simulink model "Motore_11_MM2"  (R2023b)
settings: Solver=ode23tb  StartTime=0.0  StopTime=193  FixedStep=0.001  MaxStep=1e-4  RelTol=1e-3  AbsTol=1e-2
InitFcn:
  | %Matrice=readmatrix('Profilo.csv');
  | clear
  | clc
  | 
  | m_bike=10;
  | m_driver=75;
  | mass=m_bike+m_driver;
  | a=1;
  | b=0.8;
  | h=1;
  | R=0.33;
  | 
  | load("Map.mat")
  | load("VSOC2.mat")
  | load("DriveCycle.mat")
  | t1=DriveCycle(:,1);
  | v1=DriveCycle(:,2);
  | x=length(t1);
  | t1(x)=[];
  | v1(x)=[];
  | 
  | voltage=flip(VSOC2(:,2));
  | SOC=flip(VSOC2(:,1))/100;
  | 
  | v=Map(:,1);
  | v=v*1000/3600;
  | 
  | w=v/R;
  | w=w';
  | T=Map(:,2);
  | T=T';
  | 
  | Np=1;
  | Ns=10;
  | Capacity=2; % Ah
  | 
  | k_trasm=2;
undefined symbols (not defined in the file): Map
libraries: simulink x7, slpidlib x4, autolibshared x1
settings Model: Creator=fabio  LastModifiedBy=marce
settings SolverCC: ZeroCrossAlgorithm=Adaptive
settings OptimizationCC: ReuseModelBlockBuffer=off
settings DebuggingCC: IgnoredZcDiagnostic=none

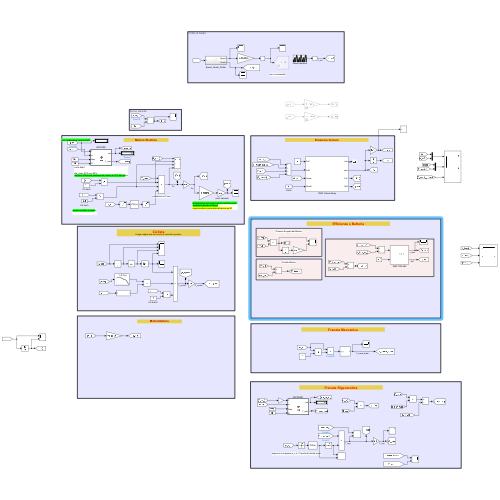
[thumbnail: Simulink's stored preview of the top-level diagram]
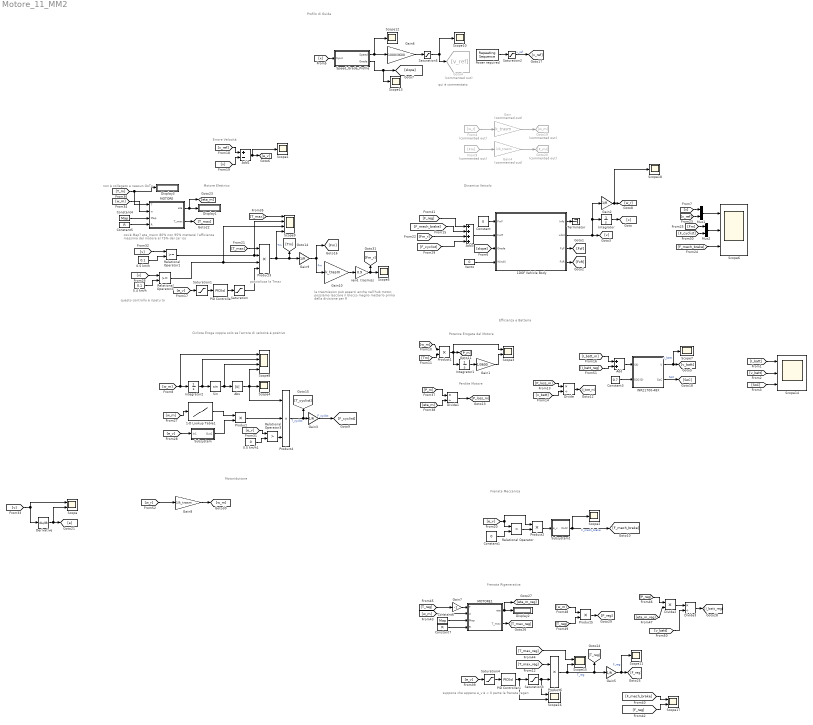
== system Motore_11_MM2 ==
  note: suppone che appena e_v è < 0 parte la frenata regen
  note: parzializza la Tmax
  note: non è collegato a neesun GoTo
  note: qui è commentato
  note: la trasmission può esserci anche nell'hub motor,
      | possiamo lasciare il blocco
      | meglio metterlo prima della divisione per R
  note: cos'è Map?
      |
      | eta_max= 80% non 95%
      | metterei l'efficienza massima del motore al 75% del car ico
  note: questo controllo è ripetu to
  note: Potenza Erogata dal Motore
  note: Motore Elettrico
  note: Profilo di Guida
  note: Errore Velocità
  note: Ciclista
      | Eroga coppia solo se l'errore di velocità è positivo
  note: Efficienza e Batteria
  note: Dinamica Veicolo
  note: Perdite Motore
  note: Frenata Rigenerativa
  note: Frenata Meccanica
  note: Motoriduttore
  " INR21700-48X" : Subsystem
      mask Display: image('C:\Users\fabio\OneDrive\Desktop\Screenshot 2023-04-19 143832.png'); % Use "Edit Image" on toolstrip to change.
  0.5 km/h : Constant  Value=0.1
  0.5 km/h1 : Constant  Value=0
  1-D Lookup Table1 : Lookup_n-D  NumberOfTableDimensions=1  BreakpointsForDimension1=w  Table=T  InternalRulePriority=Speed  RndMeth=Simplest
  1DOF Vehicle Body : Subsystem
  5.4 km/h : Constant  Value=0.1
  Abs : Abs  SaturateOnIntegerOverflow=off
  Add : Sum
  Add1 : Sum  Inputs=+-
  Add3 : Sum  Inputs=++++
  Constant : Constant  Value=0
  Constant1 : Constant  Value=0
  Constant3 : Constant  Value=0.7
  Constant4 : Constant  Value=Map
  Constant5 : Constant  Value=R
  Constant6 : Constant  Value=Map
  Constant7 : Constant  Value=R
  Derivative : Derivative
  Display1 : Display
  Display2 : Display
  Display3 : Display
  Divide : Product  Inputs=*/
  Divide1 : Product  Inputs=*/
  Divide2 : Product  Inputs=**
  Divide3 : Product  Inputs=*/
  From4 : From  Commented=on  GotoTag=w_r
  From9 : From  Commented=on  GotoTag=Fm
  Gain : Gain  Commented=on  Gain=k_trasm
  Gain1 : Gain  Gain=1/3600
  Gain10 : Gain  Gain=k_trasm
  Gain{2..3,5,9} (4 alike) : Gain  Gain=1/R
  Gain4 : Gain  Commented=on  Gain=1/k_trasm
  Gain6 : Gain  Gain=1000/3600
  Gain7 : Gain  Gain=-1
  Gain8 : Gain  Gain=1/k_trasm
  Goto19 : Goto  Commented=on  GotoTag=w_m
  Goto20 : Goto  Commented=on  GotoTag=F_mr
  Goto4 : Goto  Commented=on  GotoTag=v_ref
  Integrator : Integrator
  Integrator1 : Integrator
  Integrator2 : Integrator
  MOTORE : MATLAB Function  TreatAsAtomicUnit=on
  MOTORE1 : MATLAB Function  TreatAsAtomicUnit=on
  Mux1 : Mux  Inputs=2
  Mux2 : Mux  Inputs=2
  PID Controller : slpidlib/PID Controller  Controller=PID  Form=Parallel  TimeDomain=Continuous-time  UseExternalTs=off  SampleTime=-1  IntegratorMethod=Forward Euler  FilterMethod=Forward Euler  ControllerParametersSource=internal  P=5  I=0  UseKiTs=off  D=0  N=100  UseFilter=on  TunerSelectOption=Transfer Function Based (PID Tuner App)  InitialConditionSource=internal  InitialConditionForIntegrator=0  InitialConditionForFilter=0  DifferentiatorICPrevScaledInput=0  ExternalReset=none  TrackingMode=off  Kt=1  LimitOutput=off  SatLimitsSource=internal  UpperSaturationLimit=inf  LowerSaturationLimit=-inf  LinearizeAsGain=on  AntiWindupMode=none  Kb=1  LimitIntegrator=off  UpperIntegratorSaturationLimit=inf  LowerIntegratorSaturationLimit=-inf  POutMin=[]  POutMax=[]  IOutMin=[]  IOutMax=[]  DOutMin=[]  DOutMax=[]  NOutMin=[]  NOutMax=[]  SumOutMin=[]  SumOutMax=[]  SaturationOutMin=[]  SaturationOutMax=[]  PParamMin=[]  PParamMax=[]  IParamMin=[]  IParamMax=[]  DParamMin=[]  DParamMax=[]  NParamMin=[]  NParamMax=[]  KbParamMin=[]  KbParamMax=[]  KtParamMin=[]  KtParamMax=[]  KbOutMin=[]  KbOutMax=[]  KtOutMin=[]  KtOutMax=[]  IntegratorOutMin=[]  IntegratorOutMax=[]  FilterOutMin=[]  FilterOutMax=[]  SumI1OutMin=[]  SumI1OutMax=[]  SumI2OutMin=[]  SumI2OutMax=[]  SumI3OutMin=[]  SumI3OutMax=[]  SumI4OutMin=[]  SumI4OutMax=[]  SumDOutMin=[]  SumDOutMax=[]  DifferentiatorOutMin=[]  DifferentiatorOutMax=[]  FilterDiffOutCoefMin=[]  FilterDiffOutCoefMax=[]  ReciprocalOutMin=[]  ReciprocalOutMax=[]  SumDenOutMin=[]  SumDenOutMax=[]  SumNumOutMin=[]  SumNumOutMax=[]  DivideOutMin=[]  DivideOutMax=[]  UdiffTsProdOutMin=[]  UdiffTsProdOutMax=[]  NTsProdOutMin=[]  NTsProdOutMax=[]  UintegralTsProdOutMin=[]  UintegralTsProdOutMax=[]  UngainTsProdOutMin=[]  UngainTsProdOutMax=[]  ClampingZeroOutDataTypeStr=Inherit: Inherit via back propagation  ClampingZeroOutMin=[]  ClampingZeroOutMax=[]  FilterDenConstantOutDataTypeStr=Inherit: Inherit via back propagation  FilterDenConstantOutMin=[]  FilterDenConstantOutMax=[]  PCopyOutDataTypeStr=Inherit: Inherit via back propagation  PCopyOutMin=[]  PCopyOutMax=[]  NCopyOutDataTypeStr=Inherit: Inherit via back propagation  NCopyOutMin=[]  NCopyOutMax=[]  IntegratorContinuousStateAttributes=''  IntegratorStateMustResolveToSignalObject=off  IntegratorRTWStateStorageClass=Auto  FilterContinuousStateAttributes=''  FilterStateMustResolveToSignalObject=off  FilterRTWStateStorageClass=Auto  ParallelPVariant=InternalParameters  IdealPVariant=Disabled  IVariant=InternalParameters  DVariant=InternalParameters  IntegratorVariant=Continuous  SatVariant=Disabled  AWVariant=Passthrough  PCopyVariant=Disabled  TRVariant=Disabled  FdbkBlocksVariant=Forward  IdealPFdbkVariant=Disabled  SatFdbkVariant=Disabled  DerivativeFilterVariant=ContFilter  NVariant=InternalParameters  NCopyVariant=Disabled  FilterICVariant=InternalICsFilter  IntegratorICVariant=InternalICs  ExternalResetVariant=Disabled  TRSumVariant=Passthrough  SumFdbkVariant=Disabled  SumVariant=Sum_PID  TsampFilterVariant=InternalTs  TsampNgainVariant=Passthrough  TsampIntegralVariant=Disabled_SignalSpec  ExternalSaturationOutDataTypeStr=Inherit: Same as second input
  PID Controller1 : slpidlib/PID Controller  Controller=PID  Form=Parallel  TimeDomain=Continuous-time  UseExternalTs=off  SampleTime=-1  IntegratorMethod=Forward Euler  FilterMethod=Forward Euler  ControllerParametersSource=internal  P=5000  I=0  UseKiTs=off  D=0  N=100  UseFilter=on  TunerSelectOption=Transfer Function Based (PID Tuner App)  InitialConditionSource=internal  InitialConditionForIntegrator=0  InitialConditionForFilter=0  DifferentiatorICPrevScaledInput=0  ExternalReset=none  TrackingMode=off  Kt=1  LimitOutput=off  SatLimitsSource=internal  UpperSaturationLimit=inf  LowerSaturationLimit=-inf  LinearizeAsGain=on  AntiWindupMode=none  Kb=1  LimitIntegrator=off  UpperIntegratorSaturationLimit=inf  LowerIntegratorSaturationLimit=-inf  POutMin=[]  POutMax=[]  IOutMin=[]  IOutMax=[]  DOutMin=[]  DOutMax=[]  NOutMin=[]  NOutMax=[]  SumOutMin=[]  SumOutMax=[]  SaturationOutMin=[]  SaturationOutMax=[]  PParamMin=[]  PParamMax=[]  IParamMin=[]  IParamMax=[]  DParamMin=[]  DParamMax=[]  NParamMin=[]  NParamMax=[]  KbParamMin=[]  KbParamMax=[]  KtParamMin=[]  KtParamMax=[]  KbOutMin=[]  KbOutMax=[]  KtOutMin=[]  KtOutMax=[]  IntegratorOutMin=[]  IntegratorOutMax=[]  FilterOutMin=[]  FilterOutMax=[]  SumI1OutMin=[]  SumI1OutMax=[]  SumI2OutMin=[]  SumI2OutMax=[]  SumI3OutMin=[]  SumI3OutMax=[]  SumI4OutMin=[]  SumI4OutMax=[]  SumDOutMin=[]  SumDOutMax=[]  DifferentiatorOutMin=[]  DifferentiatorOutMax=[]  FilterDiffOutCoefMin=[]  FilterDiffOutCoefMax=[]  ReciprocalOutMin=[]  ReciprocalOutMax=[]  SumDenOutMin=[]  SumDenOutMax=[]  SumNumOutMin=[]  SumNumOutMax=[]  DivideOutMin=[]  DivideOutMax=[]  UdiffTsProdOutMin=[]  UdiffTsProdOutMax=[]  NTsProdOutMin=[]  NTsProdOutMax=[]  UintegralTsProdOutMin=[]  UintegralTsProdOutMax=[]  UngainTsProdOutMin=[]  UngainTsProdOutMax=[]  ClampingZeroOutDataTypeStr=Inherit: Inherit via back propagation  ClampingZeroOutMin=[]  ClampingZeroOutMax=[]  FilterDenConstantOutDataTypeStr=Inherit: Inherit via back propagation  FilterDenConstantOutMin=[]  FilterDenConstantOutMax=[]  PCopyOutDataTypeStr=Inherit: Inherit via back propagation  PCopyOutMin=[]  PCopyOutMax=[]  NCopyOutDataTypeStr=Inherit: Inherit via back propagation  NCopyOutMin=[]  NCopyOutMax=[]  IntegratorContinuousStateAttributes=''  IntegratorStateMustResolveToSignalObject=off  IntegratorRTWStateStorageClass=Auto  FilterContinuousStateAttributes=''  FilterStateMustResolveToSignalObject=off  FilterRTWStateStorageClass=Auto  ParallelPVariant=InternalParameters  IdealPVariant=Disabled  IVariant=InternalParameters  DVariant=InternalParameters  IntegratorVariant=Continuous  SatVariant=Disabled  AWVariant=Passthrough  PCopyVariant=Disabled  TRVariant=Disabled  FdbkBlocksVariant=Forward  IdealPFdbkVariant=Disabled  SatFdbkVariant=Disabled  DerivativeFilterVariant=ContFilter  NVariant=InternalParameters  NCopyVariant=Disabled  FilterICVariant=InternalICsFilter  IntegratorICVariant=InternalICs  ExternalResetVariant=Disabled  TRSumVariant=Passthrough  SumFdbkVariant=Disabled  SumVariant=Sum_PID  TsampFilterVariant=InternalTs  TsampNgainVariant=Passthrough  TsampIntegralVariant=Disabled_SignalSpec  ExternalSaturationOutDataTypeStr=Inherit: Same as second input
  Power required : simulink/Sources/Repeating Sequence  rep_seq_t=t1  rep_seq_y=v1
  Product{,1..2,5..6} (5 alike) : Product
  Product3 : Product  Inputs=4
  Product4 : Product  Inputs=3
  Relational Operator : RelationalOperator  Operator=<  OutDataTypeStr=boolean  RndMeth=Simplest  InputSameDT=off
  Relational Operator1 : RelationalOperator  OutDataTypeStr=boolean  RndMeth=Simplest  InputSameDT=off
  Relational Operator2 : RelationalOperator  OutDataTypeStr=boolean  RndMeth=Simplest  InputSameDT=off
  Relational Operator3 : RelationalOperator  Operator=>  OutDataTypeStr=boolean  RndMeth=Simplest  InputSameDT=off
  Saturation : Saturate  UpperLimit=1  LowerLimit=0
  Saturation1 : Saturate  UpperLimit=inf  LowerLimit=0
  Saturation2 : Saturate  UpperLimit=inf  LowerLimit=0
  Saturation3 : Saturate  UpperLimit=0  LowerLimit=-1
  Saturation4 : Saturate  UpperLimit=0  LowerLimit=-inf
  Saturation5 : Saturate  UpperLimit=inf  LowerLimit=0
  Scope{,3,15..17} (5 alike) : Scope  NumInputPorts=2
  Scope{1..2,4..5,7,10..13,18} (10 alike) : Scope
  Scope14 : Scope  NumInputPorts=3
  Scope6 : Scope  NumInputPorts=3
  Scope8 : Scope  NumInputPorts=4
  Scope9 : Scope  NumInputPorts=4
  Sin : Trigonometry
  Speed_Grade_Profile : Subsystem
  Subsystem : Subsystem
  Subsystem1 : Subsystem
  Terminator : Terminator
  Vento : Constant  Value=0
  rend. trasmiss : Gain  Gain=0.9
  wires:
  Vento/1 -> 1DOF Vehicle Body/4(WindX)
  1DOF Vehicle Body/1(Info) -> Terminator/1
  Integrator/1 -> [x]
  1DOF Vehicle Body/4(FzR) -> [FzR]
  1DOF Vehicle Body/3(FzF) -> [Fzf]
  1DOF Vehicle Body/2(xdot) -> Gain2/1, Integrator/1, [v]
  [slope] -> 1DOF Vehicle Body/3(Grade)
  Speed_Grade_Profile/2(Grade) -> Scope13/1, [slope]
  [x] -> Speed_Grade_Profile/1(Input)
  Speed_Grade_Profile/1(Speed) -> Scope12/1, Gain6/1
  Gain6/1 -> Saturation5/1
  Saturation5/1 -> Scope10/1, Goto4/1
  Add3/1 -> 1DOF Vehicle Body/2(FwR)
  [P_loss_m] -> Divide/1
  [v_batt] -> Divide/2
  Divide/1 -> [I_batt_m]
  Constant3/1 -> " INR21700-48X"/2(SOC(0))
  " INR21700-48X"/1(V) -> Scope7/1, [v_batt]  "v_batt"
  Constant/1 -> 1DOF Vehicle Body/1(FwF)
  [v] -> Add1/2
  [v_ref] -> Add1/1
  Add1/1 -> Scope1/1, [e_v]
  Constant1/1 -> Relational Operator/2
  [e_v] -> Product2/1, Relational Operator/1
  Relational Operator/1 -> Product2/2
  Product2/1 -> Subsystem1/1(e_v)
  Subsystem1/1(Out2) -> Scope2/1, [F_mech_brake]  "F_mech_brake"
  [e_v] -> Saturation1/1
  0.5 km/h/1 -> Relational Operator1/2
  Gain9/1 -> Gain10/1, [Fm]  "Fm"
  [w_m] -> Scope8/1, Integrator2/1
  Integrator2/1 -> Scope8/2, Sin/1
  Sin/1 -> Scope8/3, Abs/1
  Abs/1 -> Scope8/4, Product4/1, Scope4/1
  [v] -> Mux1/1
  Mux1/1 -> Scope6/1
  [v_ref] -> Mux1/2
  Mux2/1 -> Scope6/2
  Gain2/1 -> Scope18/1, [w_r]
  [v] -> Relational Operator2/1
  5.4 km/h/1 -> Relational Operator2/2
  Relational Operator2/1 -> Scope9/3, Product3/3
  [w_m] -> 1-D Lookup Table1/1
  1-D Lookup Table1/1 -> Product/1
  Subsystem/1(Out1) -> Product/2
  [e_v] -> Subsystem/1(In1)
  Product/1 -> Product4/2
  Product4/1 -> [T_cyclist], Gain3/1  "T_cyclist"
  Gain3/1 -> [F_cyclist]  "F_cyclist"
  [F_cyclist] -> Mux2/2
  [Fm] -> Mux2/1
  [F_mech_brake] -> Scope6/3
  Product3/1 -> Scope9/4, Gain9/1, [Tm]  "Tm"
  [e_v] -> Relational Operator3/1
  0.5 km/h1/1 -> Relational Operator3/2
  Relational Operator3/1 -> Product4/3
  Gain1/1 -> Scope3/2
  [w_m] -> Product1/1
  Product1/1 -> Scope3/1, [P_m], Integrator1/1
  [Tm] -> Product1/2
  Integrator1/1 -> Gain1/1
  [I_batt] -> Scope14/1
  [v_batt] -> Scope14/2
  " INR21700-48X"/2(SoC) -> [SoC]  "SoC"
  [SoC] -> Scope14/3
  Relational Operator1/1 -> Scope9/2, Product3/2
  From4/1 -> Gain/1
  Gain/1 -> Goto19/1
  From9/1 -> Gain4/1
  Gain4/1 -> Goto20/1
  PID Controller/1 -> Saturation/1
  [v] -> Relational Operator1/1
  Saturation1/1 -> PID Controller/1
  Saturation/1 -> Product3/4
  Power required/1 -> Saturation2/1
  Saturation2/1 -> [v_ref]  "v_ref"
  [v] -> Scope/1, Derivative/1
  Derivative/1 -> Scope/2, [a]
  [w_m] -> MOTORE/2(w)
  MOTORE/1(eta) -> [eta_m], Display1/1
  Constant4/1 -> MOTORE/3(Map)
  Constant5/1 -> MOTORE/4(R)
  MOTORE/2(T_max) -> [T_max]
  [T_max] -> Product3/1
  [T_max] -> Scope9/1
  [T_m] -> MOTORE/1(T), Display3/1
  [P_m] -> Divide1/1
  [eta_m] -> Divide1/2
  Divide1/1 -> [P_loss_m]
  Gain5/1 -> Scope11/1, [F_reg]  "F_reg"
  [T_max_reg] -> Scope15/1
  Saturation3/1 -> Scope16/1, Product6/2
  PID Controller1/1 -> Scope16/2, Saturation3/1
  [T_max_reg] -> Product6/1
  MOTORE1/2(T_max) -> [T_max_reg]
  [e_v] -> Saturation4/1
  MOTORE1/1(eta) -> [eta_m_reg], Display2/1
  Saturation4/1 -> PID Controller1/1
  [T_reg] -> Gain7/1
  Constant7/1 -> MOTORE1/4(R)
  Constant6/1 -> MOTORE1/3(Map)
  [w_m] -> MOTORE1/2(w)
  [F_cyclist] -> Add3/4
  [Fm_r] -> Add3/3
  [F_mech_brake] -> Add3/2
  [F_reg] -> Add3/1
  Product6/1 -> Scope15/2, [T_reg], Gain5/1  "T_reg"
  Gain7/1 -> MOTORE1/1(T)
  [F_mech_brake] -> Scope17/1
  [F_reg] -> Scope17/2
  Divide2/1 -> Divide3/1
  [eta_m_reg] -> Divide2/2
  [P_reg] -> Divide2/1
  Product5/1 -> [P_reg]
  [w_m] -> Product5/1
  [T_reg] -> Product5/2
  [v_batt] -> Divide3/2
  Divide3/1 -> [I_batt_reg]
  Add/1 -> " INR21700-48X"/1(I(A))
  [I_batt_m] -> Add/1
  [I_batt_reg] -> Add/2
  [w_r] -> Gain8/1
  Gain8/1 -> [w_m]
  Gain10/1 -> rend. trasmiss/1
  rend. trasmiss/1 -> [Fm_r], Scope5/1

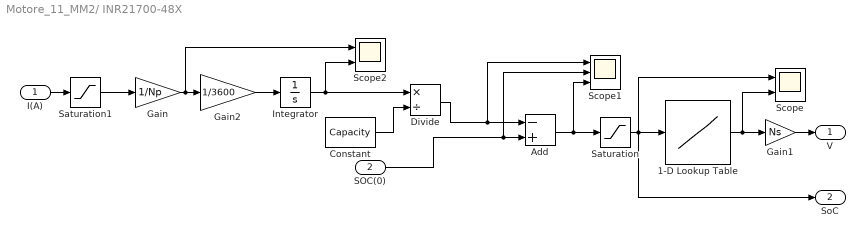
== system Motore_11_MM2/ INR21700-48X ==
  I(A) : Inport
  SOC(0) : Inport  Port=2
  1-D Lookup Table : Lookup_n-D  NumberOfTableDimensions=1  BreakpointsForDimension1=SOC  Table=voltage  InternalRulePriority=Speed  RndMeth=Simplest
  Add : Sum  Inputs=-+
  Constant : Constant  Value=Capacity
  Divide : Product  Inputs=*/
  Gain : Gain  Gain=1/Np
  Gain1 : Gain  Gain=Ns
  Gain2 : Gain  Gain=1/3600
  Integrator : Integrator
  Saturation : Saturate  UpperLimit=1  LowerLimit=0
  Saturation1 : Saturate  UpperLimit=1e6  LowerLimit=-1e6
  Scope : Scope  NumInputPorts=2
  Scope1 : Scope  NumInputPorts=3
  Scope2 : Scope  NumInputPorts=2
  V : Outport
  SoC : Outport  Port=2
  wires:
  Add/1 -> Scope1/3, Saturation/1
  I(A)/1 -> Saturation1/1
  1-D Lookup Table/1 -> Scope/2, Gain1/1
  Gain2/1 -> Integrator/1
  Saturation1/1 -> Gain/1
  Saturation/1 -> SoC/1, Scope/1, 1-D Lookup Table/1
  Gain/1 -> Gain2/1, Scope2/1
  Gain1/1 -> V/1
  Constant/1 -> Divide/2
  Integrator/1 -> Scope2/2, Divide/1
  Divide/1 -> Scope1/1, Add/1
  SOC(0)/1 -> Scope1/2, Add/2

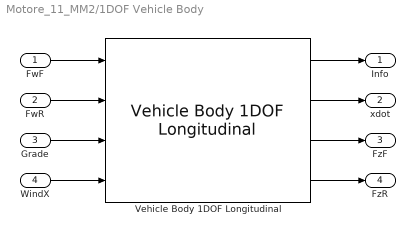
== system Motore_11_MM2/1DOF Vehicle Body ==
  FwF : Inport
  FwR : Inport  Port=2
  Grade : Inport  Port=3
  WindX : Inport  Port=4
  Vehicle Body 1DOF Longitudinal : autolibshared/Vehicle Body 1DOF Longitudinal  VariantControl=SL  extFMode=off  extMMode=off  extTamb=off  wind3D=off  aMode=2  NF=1  NR=1  m=mass  a=a  b=b  h=h  Cd=0.3  Cl=0  Cpm=0  Af=2  x_o=0  xdot_o=0  Pabs=101325  T=273  g=9.81
      settings: LibrarySourceBlock=vehdynlibeom/Vehicle Body 1DOF Longitudinal
  Info : Outport
  xdot : Outport  Port=2
  FzF : Outport  Port=3
  FzR : Outport  Port=4
  wires:
  FwF/1 -> Vehicle Body 1DOF Longitudinal/1
  FwR/1 -> Vehicle Body 1DOF Longitudinal/2
  Grade/1 -> Vehicle Body 1DOF Longitudinal/3
  WindX/1 -> Vehicle Body 1DOF Longitudinal/4
  Vehicle Body 1DOF Longitudinal/1 -> Info/1
  Vehicle Body 1DOF Longitudinal/2 -> xdot/1
  Vehicle Body 1DOF Longitudinal/3 -> FzF/1
  Vehicle Body 1DOF Longitudinal/4 -> FzR/1

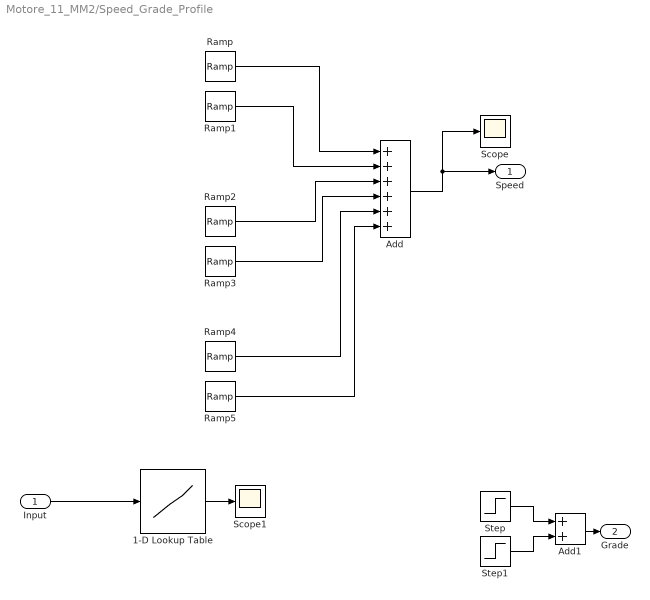
== system Motore_11_MM2/Speed_Grade_Profile ==
  Input : Inport
  1-D Lookup Table : Lookup_n-D  NumberOfTableDimensions=1  BreakpointsForDimension1=[0:0.01:3]*0.5  Table=[0:0.01:3]  InternalRulePriority=Speed  RndMeth=Simplest
  Add : Sum  Inputs=++++++
  Add1 : Sum
  Ramp : simulink/Sources/Ramp  slope=0.5  start=0  InitialOutput=0
  Ramp1 : simulink/Sources/Ramp  slope=-0.5  start=4  InitialOutput=0
  Ramp2 : simulink/Sources/Ramp  slope=1  start=7  InitialOutput=0
  Ramp3 : simulink/Sources/Ramp  slope=-1  start=10  InitialOutput=0
  Ramp4 : simulink/Sources/Ramp  slope=-2  start=15  InitialOutput=0
  Ramp5 : simulink/Sources/Ramp  slope=1  start=20  InitialOutput=0
  Scope : Scope
  Scope1 : Scope
  Step : Step  Time=12  After=5  SampleTime=0
  Step1 : Step  Time=17.5  After=-5  SampleTime=0
  Speed : Outport
  Grade : Outport  Port=2
  wires:
  Ramp/1 -> Add/1
  Ramp1/1 -> Add/2
  Ramp2/1 -> Add/3
  Ramp3/1 -> Add/4
  Add/1 -> Scope/1, Speed/1
  Input/1 -> 1-D Lookup Table/1
  1-D Lookup Table/1 -> Scope1/1
  Ramp4/1 -> Add/5
  Ramp5/1 -> Add/6
  Add1/1 -> Grade/1
  Step1/1 -> Add1/2
  Step/1 -> Add1/1

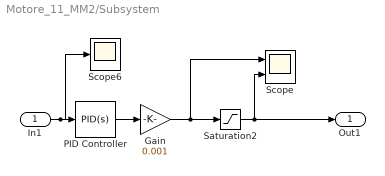
== system Motore_11_MM2/Subsystem ==
  In1 : Inport
  Gain : Gain  Gain=0.001
  PID Controller : slpidlib/PID Controller  Controller=PID  Form=Parallel  TimeDomain=Continuous-time  UseExternalTs=off  SampleTime=-1  IntegratorMethod=Forward Euler  FilterMethod=Forward Euler  ControllerParametersSource=internal  P=10000  I=0.01  UseKiTs=off  D=0  N=100  UseFilter=on  TunerSelectOption=Transfer Function Based (PID Tuner App)  InitialConditionSource=internal  InitialConditionForIntegrator=0  InitialConditionForFilter=0  DifferentiatorICPrevScaledInput=0  ExternalReset=none  TrackingMode=off  Kt=1  LimitOutput=off  SatLimitsSource=internal  UpperSaturationLimit=inf  LowerSaturationLimit=-inf  LinearizeAsGain=off  AntiWindupMode=none  Kb=1  LimitIntegrator=off  UpperIntegratorSaturationLimit=inf  LowerIntegratorSaturationLimit=-inf  POutMin=[]  POutMax=[]  IOutMin=[]  IOutMax=[]  DOutMin=[]  DOutMax=[]  NOutMin=[]  NOutMax=[]  SumOutMin=[]  SumOutMax=[]  SaturationOutMin=[]  SaturationOutMax=[]  PParamMin=[]  PParamMax=[]  IParamMin=[]  IParamMax=[]  DParamMin=[]  DParamMax=[]  NParamMin=[]  NParamMax=[]  KbParamMin=[]  KbParamMax=[]  KtParamMin=[]  KtParamMax=[]  KbOutMin=[]  KbOutMax=[]  KtOutMin=[]  KtOutMax=[]  IntegratorOutMin=[]  IntegratorOutMax=[]  FilterOutMin=[]  FilterOutMax=[]  SumI1OutMin=[]  SumI1OutMax=[]  SumI2OutMin=[]  SumI2OutMax=[]  SumI3OutMin=[]  SumI3OutMax=[]  SumI4OutMin=[]  SumI4OutMax=[]  SumDOutMin=[]  SumDOutMax=[]  DifferentiatorOutMin=[]  DifferentiatorOutMax=[]  FilterDiffOutCoefMin=[]  FilterDiffOutCoefMax=[]  ReciprocalOutMin=[]  ReciprocalOutMax=[]  SumDenOutMin=[]  SumDenOutMax=[]  SumNumOutMin=[]  SumNumOutMax=[]  DivideOutMin=[]  DivideOutMax=[]  UdiffTsProdOutMin=[]  UdiffTsProdOutMax=[]  NTsProdOutMin=[]  NTsProdOutMax=[]  UintegralTsProdOutMin=[]  UintegralTsProdOutMax=[]  UngainTsProdOutMin=[]  UngainTsProdOutMax=[]  ClampingZeroOutDataTypeStr=Inherit: Inherit via back propagation  ClampingZeroOutMin=[]  ClampingZeroOutMax=[]  FilterDenConstantOutDataTypeStr=Inherit: Inherit via back propagation  FilterDenConstantOutMin=[]  FilterDenConstantOutMax=[]  PCopyOutDataTypeStr=Inherit: Inherit via back propagation  PCopyOutMin=[]  PCopyOutMax=[]  NCopyOutDataTypeStr=Inherit: Inherit via back propagation  NCopyOutMin=[]  NCopyOutMax=[]  IntegratorContinuousStateAttributes=''  IntegratorStateMustResolveToSignalObject=off  IntegratorRTWStateStorageClass=Auto  FilterContinuousStateAttributes=''  FilterStateMustResolveToSignalObject=off  FilterRTWStateStorageClass=Auto  ParallelPVariant=InternalParameters  IdealPVariant=Disabled  IVariant=InternalParameters  DVariant=InternalParameters  IntegratorVariant=Continuous  SatVariant=Disabled  AWVariant=Passthrough  PCopyVariant=Disabled  TRVariant=Disabled  FdbkBlocksVariant=Forward  IdealPFdbkVariant=Disabled  SatFdbkVariant=Disabled  DerivativeFilterVariant=ContFilter  NVariant=InternalParameters  NCopyVariant=Disabled  FilterICVariant=InternalICsFilter  IntegratorICVariant=InternalICs  ExternalResetVariant=Disabled  TRSumVariant=Passthrough  SumFdbkVariant=Disabled  SumVariant=Sum_PID  TsampFilterVariant=InternalTs  TsampNgainVariant=Passthrough  TsampIntegralVariant=Disabled_SignalSpec  ExternalSaturationOutDataTypeStr=Inherit: Same as second input
  Saturation2 : Saturate  UpperLimit=1  LowerLimit=0
  Scope : Scope  NumInputPorts=2
  Scope6 : Scope
  Out1 : Outport
  wires:
  In1/1 -> Scope6/1, PID Controller/1
  Saturation2/1 -> Scope/2, Out1/1
  PID Controller/1 -> Gain/1
  Gain/1 -> Scope/1, Saturation2/1

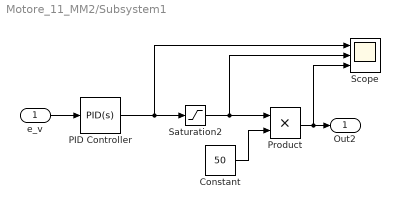
== system Motore_11_MM2/Subsystem1 ==
  e_v : Inport
  Constant : Constant  Value=50
  PID Controller : slpidlib/PID Controller  Controller=PID  Form=Parallel  TimeDomain=Continuous-time  UseExternalTs=off  SampleTime=-1  IntegratorMethod=Forward Euler  FilterMethod=Forward Euler  ControllerParametersSource=internal  P=10000  I=0.01  UseKiTs=off  D=0  N=100  UseFilter=on  TunerSelectOption=Transfer Function Based (PID Tuner App)  InitialConditionSource=internal  InitialConditionForIntegrator=0  InitialConditionForFilter=0  DifferentiatorICPrevScaledInput=0  ExternalReset=none  TrackingMode=off  Kt=1  LimitOutput=off  SatLimitsSource=internal  UpperSaturationLimit=inf  LowerSaturationLimit=-inf  LinearizeAsGain=on  AntiWindupMode=none  Kb=1  LimitIntegrator=off  UpperIntegratorSaturationLimit=inf  LowerIntegratorSaturationLimit=-inf  POutMin=[]  POutMax=[]  IOutMin=[]  IOutMax=[]  DOutMin=[]  DOutMax=[]  NOutMin=[]  NOutMax=[]  SumOutMin=[]  SumOutMax=[]  SaturationOutMin=[]  SaturationOutMax=[]  PParamMin=[]  PParamMax=[]  IParamMin=[]  IParamMax=[]  DParamMin=[]  DParamMax=[]  NParamMin=[]  NParamMax=[]  KbParamMin=[]  KbParamMax=[]  KtParamMin=[]  KtParamMax=[]  KbOutMin=[]  KbOutMax=[]  KtOutMin=[]  KtOutMax=[]  IntegratorOutMin=[]  IntegratorOutMax=[]  FilterOutMin=[]  FilterOutMax=[]  SumI1OutMin=[]  SumI1OutMax=[]  SumI2OutMin=[]  SumI2OutMax=[]  SumI3OutMin=[]  SumI3OutMax=[]  SumI4OutMin=[]  SumI4OutMax=[]  SumDOutMin=[]  SumDOutMax=[]  DifferentiatorOutMin=[]  DifferentiatorOutMax=[]  FilterDiffOutCoefMin=[]  FilterDiffOutCoefMax=[]  ReciprocalOutMin=[]  ReciprocalOutMax=[]  SumDenOutMin=[]  SumDenOutMax=[]  SumNumOutMin=[]  SumNumOutMax=[]  DivideOutMin=[]  DivideOutMax=[]  UdiffTsProdOutMin=[]  UdiffTsProdOutMax=[]  NTsProdOutMin=[]  NTsProdOutMax=[]  UintegralTsProdOutMin=[]  UintegralTsProdOutMax=[]  UngainTsProdOutMin=[]  UngainTsProdOutMax=[]  ClampingZeroOutDataTypeStr=Inherit: Inherit via back propagation  ClampingZeroOutMin=[]  ClampingZeroOutMax=[]  FilterDenConstantOutDataTypeStr=Inherit: Inherit via back propagation  FilterDenConstantOutMin=[]  FilterDenConstantOutMax=[]  PCopyOutDataTypeStr=Inherit: Inherit via back propagation  PCopyOutMin=[]  PCopyOutMax=[]  NCopyOutDataTypeStr=Inherit: Inherit via back propagation  NCopyOutMin=[]  NCopyOutMax=[]  IntegratorContinuousStateAttributes=''  IntegratorStateMustResolveToSignalObject=off  IntegratorRTWStateStorageClass=Auto  FilterContinuousStateAttributes=''  FilterStateMustResolveToSignalObject=off  FilterRTWStateStorageClass=Auto  ParallelPVariant=InternalParameters  IdealPVariant=Disabled  IVariant=InternalParameters  DVariant=InternalParameters  IntegratorVariant=Continuous  SatVariant=Disabled  AWVariant=Passthrough  PCopyVariant=Disabled  TRVariant=Disabled  FdbkBlocksVariant=Forward  IdealPFdbkVariant=Disabled  SatFdbkVariant=Disabled  DerivativeFilterVariant=ContFilter  NVariant=InternalParameters  NCopyVariant=Disabled  FilterICVariant=InternalICsFilter  IntegratorICVariant=InternalICs  ExternalResetVariant=Disabled  TRSumVariant=Passthrough  SumFdbkVariant=Disabled  SumVariant=Sum_PID  TsampFilterVariant=InternalTs  TsampNgainVariant=Passthrough  TsampIntegralVariant=Disabled_SignalSpec  ExternalSaturationOutDataTypeStr=Inherit: Same as second input
  Product : Product
  Saturation2 : Saturate  UpperLimit=0  LowerLimit=-1
  Scope : Scope  NumInputPorts=3
  Out2 : Outport
  wires:
  e_v/1 -> PID Controller/1
  PID Controller/1 -> Saturation2/1, Scope/1
  Saturation2/1 -> Product/1, Scope/2
  Product/1 -> Scope/3, Out2/1
  Constant/1 -> Product/2

== matlab function Motore_11_MM2/MOTORE1 ==
  data: T input; eta output; w input; T_max output; Map input; R input
function [eta, T_max] = fcn(T, w, Map, R)

v=Map(:,1);
v=v*1000/3600;

w_n=v/R;
w_n=w_n';
T_n=Map(:,2);
T_n=T_n';

% Dato w, individua la velocità angolare più vicina nella mappa
differenza_assoluta = abs(w_n - w);
[~, indice_minimo] = min(differenza_assoluta);
posizione_piu_vicina = indice_minimo;


% Crea un vettore di efficienza con valore massimo nel valore medio
eta_max = 0.95; % Efficienza massima
eta_min = 0.5;  % Efficienza minima
risoluzione = 101; % Grandezza del vettore eta
indice_centrale = ceil(risoluzione / 2); % Calcola l'indice centrale
eta_distr = linspace(eta_min, eta_max, risoluzione); % Creazione del vettore eta
eta_distr = circshift(eta_distr, [0, indice_centrale - 1]); % Sposta l'efficienza massima al centro del vettore
eta_distr = eta_max - abs(linspace(-1, 1, risoluzione)).*(eta_max - eta_min); % Calcola l'andamento continuo dell'efficienza

T_max=T_n(posizione_piu_vicina);
T_min=0;
T_vect = linspace(0, T_max, risoluzione);
differenza_assoluta = abs(T_vect - T);
[~, indice_minimo] = min(differenza_assoluta);
posizione_piu_vicina = indice_minimo;
eta=eta_distr(posizione_piu_vicina);

end

== matlab function Motore_11_MM2/MOTORE ==
  data: T input; eta output; w input; T_max output; Map input; R input
function [eta, T_max] = fcn(T, w, Map, R)

v=Map(:,1);
v=v*1000/3600;

w_n=v/R;
w_n=w_n';
T_n=Map(:,2);
T_n=T_n';

% Dato w, individua la velocità angolare più vicina nella mappa
differenza_assoluta = abs(w_n - w);
[~, indice_minimo] = min(differenza_assoluta);
posizione_piu_vicina = indice_minimo;


% Crea un vettore di efficienza con valore massimo nel valore medio
eta_max = 0.95; % Efficienza massima
eta_min = 0.5;  % Efficienza minima
risoluzione = 101; % Grandezza del vettore eta
indice_centrale = ceil(risoluzione / 2); % Calcola l'indice centrale
eta_distr = linspace(eta_min, eta_max, risoluzione); % Creazione del vettore eta
eta_distr = circshift(eta_distr, [0, indice_centrale - 1]); % Sposta l'efficienza massima al centro del vettore
eta_distr = eta_max - abs(linspace(-1, 1, risoluzione)).*(eta_max - eta_min); % Calcola l'andamento continuo dell'efficienza

T_max=T_n(posizione_piu_vicina);
T_min=0;
T_vect = linspace(0, T_max, risoluzione);
differenza_assoluta = abs(T_vect - T);
[~, indice_minimo] = min(differenza_assoluta);
posizione_piu_vicina = indice_minimo;
eta=eta_distr(posizione_piu_vicina);

end
